simulink model "sensivity"  (Simulink 7.7)
settings: Solver=ode45  StartTime=0.0  StopTime=10  RelTol=1e-3
settings Model: Creator=spu  LastModifiedBy=mestan

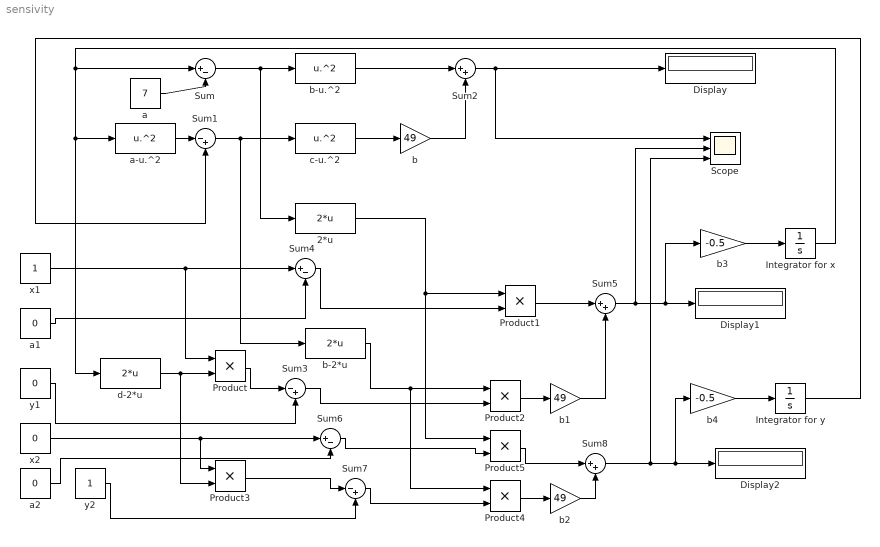
== system sensivity ==
  2*u : MATLABFcn  MATLABFcn=2*u
  Display : Display
  Display1 : Display
  Display2 : Display
  Integrator for x : Integrator  InitialCondition=2
  Integrator for y : Integrator  InitialCondition=2
  Product{,1..5} (6 alike) : Product  RndMeth=Zero
  Scope : Scope  NumInputPorts=3
      settings: YMin=15.25~1.5~-2.3  YMax=17.75~6.5~-1.7
  Sum : Sum  Inputs=|+-
  Sum1 : Sum  Inputs=|-+
  Sum2 : Sum  Inputs=|++
  Sum3 : Sum  Inputs=|-+
  Sum4 : Sum  Inputs=|+-
  Sum5 : Sum  Inputs=|++
  Sum6 : Sum  Inputs=|+-
  Sum7 : Sum  Inputs=|-+
  Sum8 : Sum  Inputs=|++
  a : Constant  Value=7
  a-u.^2 : MATLABFcn  MATLABFcn=u.^2
  a1 : Constant  Value=0
  a2 : Constant  Value=0
  b : Gain  Gain=49
  b-2*u : MATLABFcn  MATLABFcn=2*u
  b-u.^2 : MATLABFcn  MATLABFcn=u.^2
  b1 : Gain  Gain=49
  b2 : Gain  Gain=49
  b3 : Gain  Gain=-0.5
  b4 : Gain  Gain=-0.5
  c-u.^2 : MATLABFcn  MATLABFcn=u.^2
  d-2*u : MATLABFcn  MATLABFcn=2*u
  x1 : Constant
  x2 : Constant  Value=0
  y1 : Constant  Value=0
  y2 : Constant
  wires:
  Sum/1 -> b-u.^2/1, 2*u/1
  Sum1/1 -> c-u.^2/1, b-2*u/1
  c-u.^2/1 -> b/1
  b-u.^2/1 -> Sum2/1
  b/1 -> Sum2/2
  a-u.^2/1 -> Sum1/1
  Sum2/1 -> Scope/1, Display/1
  a/1 -> Sum/2
  x1/1 -> Product/1, Sum4/1
  d-2*u/1 -> Product3/2, Product/2
  Product/1 -> Sum3/1
  y1/1 -> Sum3/2
  a1/1 -> Sum4/2
  Sum4/1 -> Product1/2
  2*u/1 -> Product5/1, Product1/1
  Sum3/1 -> Product2/2
  b-2*u/1 -> Product2/1, Product4/1
  Product2/1 -> b1/1
  Product1/1 -> Sum5/1
  b1/1 -> Sum5/2
  Sum5/1 -> Scope/2, Display1/1, b3/1
  a2/1 -> Sum6/2
  x2/1 -> Sum6/1, Product3/1
  Product3/1 -> Sum7/1
  y2/1 -> Sum7/2
  Sum7/1 -> Product4/2
  Sum6/1 -> Product5/2
  Product5/1 -> Sum8/1
  Product4/1 -> b2/1
  Sum8/1 -> b4/1, Display2/1, Scope/3
  b2/1 -> Sum8/2
  b3/1 -> Integrator for x/1
  b4/1 -> Integrator for y/1
  Integrator for x/1 -> Sum/1, d-2*u/1, a-u.^2/1
  Integrator for y/1 -> Sum1/2
